simulink model "kapitza_manual"  (R2025b)
settings: Solver=ode45  StartTime=0.0  StopTime=100  MaxStep=1/(100*f)  RelTol=1e-7  AbsTol=1e-9
values from neighbouring files (symbols this model uses):
  p = [g; l; m; b; A; f]    [parameters_kapitza.m]
  x0 = [75*pi/180; 0]    [parameters_kapitza.m]
settings Model: Creator=rafae  LastModifiedBy=rafae
settings SolverCC: AutoScaleAbsTol=off

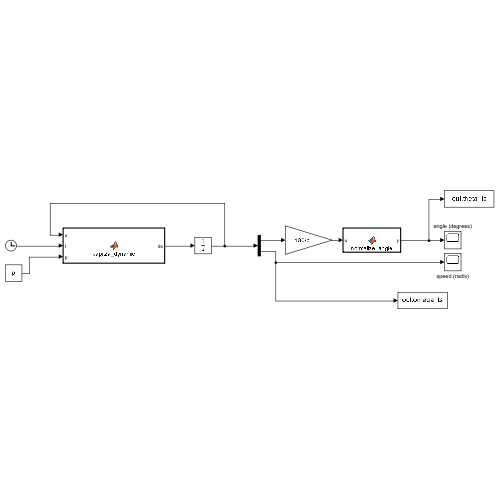
[thumbnail: Simulink's stored preview of the top-level diagram]
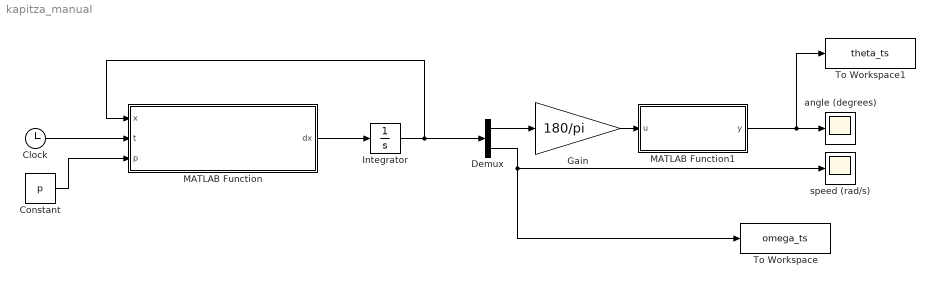
== system kapitza_manual ==
  Clock : Clock
  Constant : Constant  Value=p
  Demux : Demux  Outputs=2
  Gain : Gain  Gain=180/pi
  Integrator : Integrator  InitialCondition=x0
  MATLAB Function : MATLAB Function  TreatAsAtomicUnit=on
  MATLAB Function1 : MATLAB Function  TreatAsAtomicUnit=on
  To Workspace : ToWorkspace  VariableName=omega_ts  SaveFormat=Timeseries  SampleTime=-1
  To Workspace1 : ToWorkspace  VariableName=theta_ts  SaveFormat=Timeseries  SampleTime=-1
  angle (degrees) : Scope
      settings: ActiveDisplayYMinimum=-1  ActiveDisplayYMaximum=1
  speed (rad/s) : Scope
      settings: ActiveDisplayYMinimum=-1  ActiveDisplayYMaximum=1
  wires:
  Clock/1 -> MATLAB Function/2(t)
  Constant/1 -> MATLAB Function/3(p)
  MATLAB Function/1(dx) -> Integrator/1
  Integrator/1 -> MATLAB Function/1(x), Demux/1
  Demux/2 -> speed (rad/s)/1, To Workspace/1
  Gain/1 -> MATLAB Function1/1(u)
  Demux/1 -> Gain/1
  MATLAB Function1/1(y) -> To Workspace1/1, angle (degrees)/1

== matlab function kapitza_manual/MATLAB Function ==
  data: x input; dx output; t input; p input
function dx = kapitza_dynamic(x, t, p)

g = p(1);
l = p(2);
m = p(3);
b = p(4);
A = p(5);
f = p(6);

theta = x(1);
omega = x(2);

Omega = 2*pi*f;


vv = A*Omega*sin(Omega*t);
av = A*Omega^2*cos(Omega*t);

dx = zeros(2,1);

dx(1) = omega;

dx(2) = (g/l)*sin(theta) ...
      - (b/m)*omega ...
      + (b/(m*l))*vv*sin(theta) ...
      - (av/l)*sin(theta);
end

== matlab function kapitza_manual/MATLAB Function1 ==
  data: u input; y output
function y = normalize_angle(u)
    y = mod(u + 180, 360) - 180;
end
